simulink model "One_Stage"  (R2021b)
settings: Solver=VariableStepAuto  StartTime=0.0  StopTime=10.0  RelTol=1e-3
settings Model: Creator=Personal  LastModifiedBy=Personal

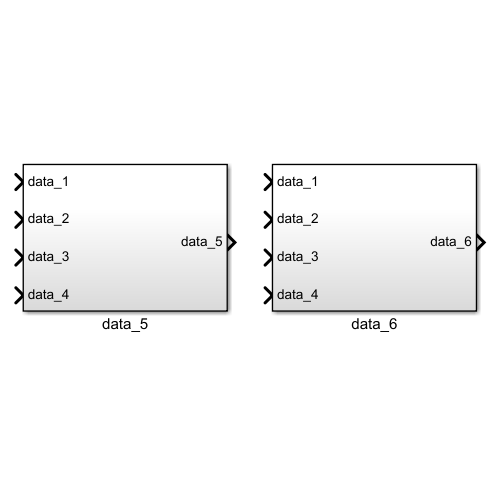
[thumbnail: Simulink's stored preview of the top-level diagram]
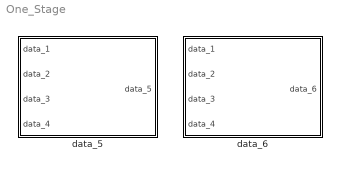
== system One_Stage ==
  data_5 : Subsystem
  data_6 : Subsystem

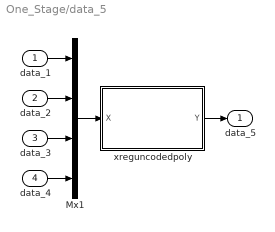
== system One_Stage/data_5 ==
  data_1 : Inport
  data_2 : Inport  Port=2
  data_3 : Inport  Port=3
  data_4 : Inport  Port=4
  Mx1 : Mux
  xreguncodedpoly : Subsystem
      mask init:
      | xregmaskinitialization;
  data_5 : Outport
  wires:
  data_1/1 -> Mx1/1
  data_2/1 -> Mx1/2
  data_3/1 -> Mx1/3
  data_4/1 -> Mx1/4
  Mx1/1 -> xreguncodedpoly/1(X)
  xreguncodedpoly/1(Y) -> data_5/1

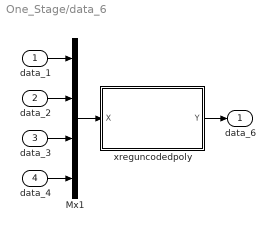
== system One_Stage/data_6 ==
  data_1 : Inport
  data_2 : Inport  Port=2
  data_3 : Inport  Port=3
  data_4 : Inport  Port=4
  Mx1 : Mux
  xreguncodedpoly : Subsystem
      mask init:
      | xregmaskinitialization;
  data_6 : Outport
  wires:
  data_1/1 -> Mx1/1
  data_2/1 -> Mx1/2
  data_3/1 -> Mx1/3
  data_4/1 -> Mx1/4
  Mx1/1 -> xreguncodedpoly/1(X)
  xreguncodedpoly/1(Y) -> data_6/1

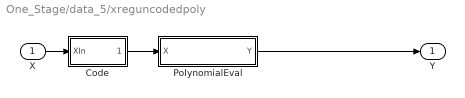
== system One_Stage/data_5/xreguncodedpoly ==
  X : Inport
  Code : Subsystem
  PolynomialEval : Subsystem
  Y : Outport
  wires:
  X/1 -> Code/1(XIn)
  Code/1(XCoded) -> PolynomialEval/1(X)
  PolynomialEval/1(Y) -> Y/1

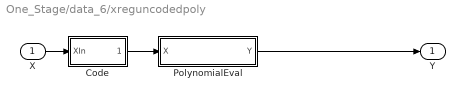
== system One_Stage/data_6/xreguncodedpoly ==
  X : Inport
  Code : Subsystem
  PolynomialEval : Subsystem
  Y : Outport
  wires:
  X/1 -> Code/1(XIn)
  Code/1(XCoded) -> PolynomialEval/1(X)
  PolynomialEval/1(Y) -> Y/1

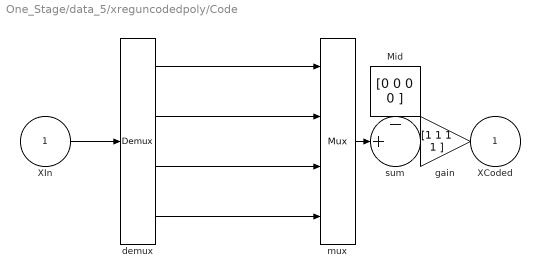
== system One_Stage/data_5/xreguncodedpoly/Code ==
  XIn : Inport
  Mid : Constant  Value=[0 0 0 0 ]
  demux : Demux
  gain : Gain  Gain=[1 1 1 1 ]
  mux : Mux
  sum : Sum  Inputs=-+|
  XCoded : Outport
  wires:
  demux/1 -> mux/1
  demux/2 -> mux/2
  demux/3 -> mux/3
  demux/4 -> mux/4
  Mid/1 -> sum/1
  XIn/1 -> demux/1
  mux/1 -> sum/2
  sum/1 -> gain/1
  gain/1 -> XCoded/1

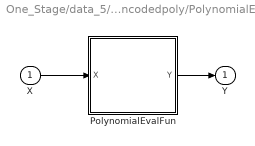
== system One_Stage/data_5/xreguncodedpoly/PolynomialEval ==
  X : Inport
  PolynomialEvalFun : MATLAB Function  TreatAsAtomicUnit=on
  Y : Outport
  wires:
  X/1 -> PolynomialEvalFun/1(X)
  PolynomialEvalFun/1(Y) -> Y/1

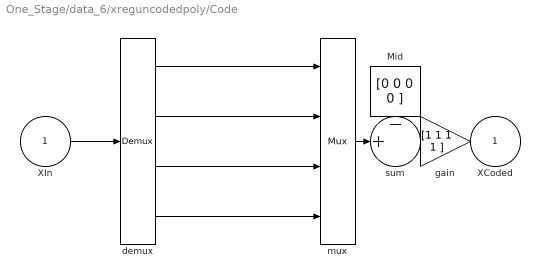
== system One_Stage/data_6/xreguncodedpoly/Code ==
  XIn : Inport
  Mid : Constant  Value=[0 0 0 0 ]
  demux : Demux
  gain : Gain  Gain=[1 1 1 1 ]
  mux : Mux
  sum : Sum  Inputs=-+|
  XCoded : Outport
  wires:
  demux/1 -> mux/1
  demux/2 -> mux/2
  demux/3 -> mux/3
  demux/4 -> mux/4
  Mid/1 -> sum/1
  XIn/1 -> demux/1
  mux/1 -> sum/2
  sum/1 -> gain/1
  gain/1 -> XCoded/1

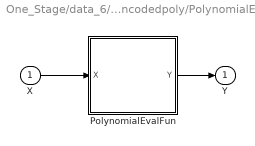
== system One_Stage/data_6/xreguncodedpoly/PolynomialEval ==
  X : Inport
  PolynomialEvalFun : MATLAB Function  TreatAsAtomicUnit=on
  Y : Outport
  wires:
  X/1 -> PolynomialEvalFun/1(X)
  PolynomialEvalFun/1(Y) -> Y/1

== matlab function One_Stage/data_6/xreguncodedpoly/PolynomialEval/PolynomialEvalFun ==
  data: X input size=nfactors; Y output; coeffs parameter
function Y = fcn(X, coeffs)
%#codegen

% This function specifies a polynomial with 4 inputs: 
% 	TR	 = order 3
% 	A	 = order 3
% 	L	 = order 2
% 	T	 = order 2
% Maximum interaction order = 3
%
% The model definition is:
% -5498.3094 - 766.83107*TR + 549.31751*A - 44.711683*L - 2.1149066*T +   
% 3.5641621*TR^2 + 0.0049845809*TR*A + 0.097951231*TR*L - 74.970231*TR*T +
% 82.339876*A^2 - 0.55545038*A*L + 0.001290913*A*T - 0.0019350527*L^2 -   
% 2.031822*L*T - 1.6766583*T^2 + 0.0013545002*TR^3 + 0.2568036*TR^2*A +   
% 1945.2757*TR*A^2 - 199.82438*A^3                                        

% Autogenerated by the Model-Based Calibration Toolbox on 26-Oct-2022 10:56:09.

Y = coeffs(1);
Y = Y + X(1)*(coeffs(2) + X(1)*(coeffs(3) + X(1)*coeffs(4) + X(2)*coeffs(5)) + X(2)*(coeffs(6) + X(2)*coeffs(7)) + X(3)*(coeffs(8)) + X(4)*(coeffs(9)));
Y = Y + X(2)*(coeffs(10) + X(2)*(coeffs(11) + X(2)*coeffs(12)) + X(3)*(coeffs(13)) + X(4)*(coeffs(14)));
Y = Y + X(3)*(coeffs(15) + X(3)*(coeffs(16)) + X(4)*(coeffs(17)));
Y = Y + X(4)*(coeffs(18) + X(4)*(coeffs(19)));

== matlab function One_Stage/data_5/xreguncodedpoly/PolynomialEval/PolynomialEvalFun ==
  data: X input size=nfactors; Y output; coeffs parameter
function Y = fcn(X, coeffs)
%#codegen

% This function specifies a polynomial with 4 inputs: 
% 	TR	 = order 3
% 	A	 = order 3
% 	L	 = order 2
% 	T	 = order 2
% Maximum interaction order = 3
%
% The model definition is:
% -633.36 - 58.95065*TR + 1.34878*A + 0.7781926*L + 0.1083333*T - 0.3090848*TR^2 -
% 0.00138335*TR*A + 0.01947693*TR*L + 0.01493413*TR*T + 18.90003*A^2 -            
% 0.1397954*A*L + 0.0003588797*A*T + 0.0007922034*L^2 + 0.0005149436*L*T -        
% 0.1245315*T^2 - 4.443121e-05*TR^3 - 0.0002890329*TR^2*A + 0.0880576*TR*A^2 -    
% 0.01253483*A^3                                                                  

% Autogenerated by the Model-Based Calibration Toolbox on 26-Oct-2022 10:56:06.

Y = coeffs(1);
Y = Y + X(1)*(coeffs(2) + X(1)*(coeffs(3) + X(1)*coeffs(4) + X(2)*coeffs(5)) + X(2)*(coeffs(6) + X(2)*coeffs(7)) + X(3)*(coeffs(8)) + X(4)*(coeffs(9)));
Y = Y + X(2)*(coeffs(10) + X(2)*(coeffs(11) + X(2)*coeffs(12)) + X(3)*(coeffs(13)) + X(4)*(coeffs(14)));
Y = Y + X(3)*(coeffs(15) + X(3)*(coeffs(16)) + X(4)*(coeffs(17)));
Y = Y + X(4)*(coeffs(18) + X(4)*(coeffs(19)));
